simulink model "flexibleBeamILCBF"  (R2021a)
settings: Solver=ode23t  StartTime=0.0  StopTime=Tend  FixedStep=Ts  RelTol=1e-2
values from neighbouring files (symbols this model uses):
  G = G+2*(Cm(r)*Bm(r))/(s^2+2*zeta(r-1)*wn(r-1)*s+wn(r-1)^2)    [ModelFlexibleBeamFirstPrinciple.m]
  l = 500    [FRFSimscape.m]    (also in GPSnap.m; dataSetGPSnap_10092021.mat; dataSetGPSnap_10092021_2.mat)
  POI = 250    [FRFSimscape.m]
  Ts = 5e-4    (= 0.0005)    [FRFSimscape.m]    (also in GPSnap.m = 0.001; ILCBFSimscape.m = 0.001)
libraries: dspsrcs4 x2, simulink x1
settings Model: Creator=s152009  LastModifiedBy=s152009

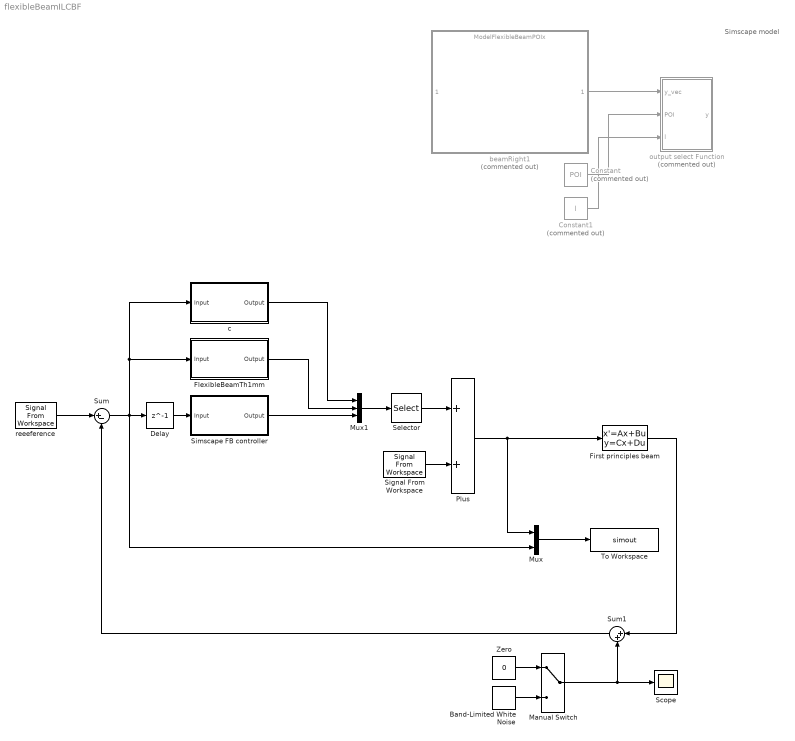
== system flexibleBeamILCBF ==
  note: Simscape model
  Band-Limited White Noise : simulink/Sources/Band-Limited White Noise  Cov=[1e-16]  Ts=Ts  seed=[23341]
  Constant : Constant  Commented=on  Value=POI
  Constant1 : Constant  Commented=on  Value=l
  Delay : Delay  DelayLength=1
  First principles beam : StateSpace  A=G.A  B=G.B  C=G.C  D=G.D  InitialCondition=0
  FlexibleBeamTh1mm : Subsystem
  Manual Switch : ManualSwitch
  Mux : Mux  Inputs=2
  Mux1 : Mux  Inputs=3
  Plus : Sum
  Scope : Scope
  Selector : Selector  InputPortWidth=3  IndexOptions=Index vector (dialog)  Indices=[1]  OutputSizes=1
  Signal From Workspace : dspsrcs4/Signal From Workspace  X=f_j  Ts=Ts  nsamps=1  OutputAfterFinalValue=Setting to zero  ignoreOrWarnInputAndFrameLengths=off  OutputFrames=off
  Simscape FB controller : Subsystem
  Sum : Sum  Inputs=|+-
  Sum1 : Sum  Inputs=|++
  To Workspace : ToWorkspace  VariableName=simout  SampleTime=Ts
  Zero : Constant  Value=0  OutDataTypeStr=Inherit: Inherit via back propagation
  beamRight1 : ModelReference  Commented=on  ModelNameDialog=ModelFlexibleBeamPOIx.slx  SimulationMode=Normal  ModelReferenceVersion=1.15
  c : Subsystem
  output select Function : MATLAB Function  Commented=on  TreatAsAtomicUnit=on
  reeeference : dspsrcs4/Signal From Workspace  X=r  Ts=Ts  nsamps=1  OutputAfterFinalValue=Holding final value  ignoreOrWarnInputAndFrameLengths=off  OutputFrames=off
  wires:
  reeeference/1 -> Sum/1
  Signal From Workspace/1 -> Plus/2
  Plus/1 -> First principles beam/1, Mux/1
  Sum/1 -> Mux/2, Delay/1, c/1(Input), FlexibleBeamTh1mm/1(Input)
  Mux/1 -> To Workspace/1
  Constant/1 -> output select Function/2(POI)
  Constant1/1 -> output select Function/3(l)
  Selector/1 -> Plus/1
  Simscape FB controller/1(Output) -> Mux1/3
  Delay/1 -> Simscape FB controller/1(Input)
  Mux1/1 -> Selector/1
  beamRight1/1 -> output select Function/1(y_vec)
  FlexibleBeamTh1mm/1(Output) -> Mux1/2
  First principles beam/1 -> Sum1/1
  Sum1/1 -> Sum/2
  Manual Switch/1 -> Scope/1, Sum1/2
  Zero/1 -> Manual Switch/1
  Band-Limited White Noise/1 -> Manual Switch/2
  c/1(Output) -> Mux1/1

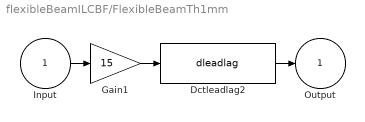
== system flexibleBeamILCBF/FlexibleBeamTh1mm ==
  Input : Inport
  Dctleadlag2 : S-Function  FunctionName=dleadlag  Parameters=f_num, f_den, 0.001  SFunctionDeploymentMode=off  EnableBusSupport=off  mask(dctools){f_num=0.5, f_den=5}
      mask prompts: f_num "Zero [Hz]"; f_den "Pole [Hz]"
      mask help: This block implements a discrete time leadlag filter.
      mask Display: disp('DCT leadlag')
  Gain1 : Gain  Gain=15
  Output : Outport
  wires:
  Input/1 -> Gain1/1
  Gain1/1 -> Dctleadlag2/1
  Dctleadlag2/1 -> Output/1

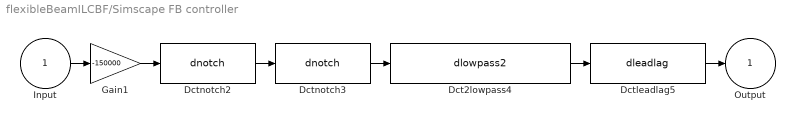
== system flexibleBeamILCBF/Simscape FB controller ==
  Input : Inport
  Dct2lowpass4 : S-Function  FunctionName=dlowpass2  Parameters=f_den, b_den, 0.001  SFunctionDeploymentMode=off  EnableBusSupport=off  mask(dctools){f_den=10, b_den=0.7}
      mask prompts: f_den "Pole [Hz]"; b_den "Damping pole [-]"
      mask help: This block implements a discrete time 2nd order lowpass filter.
      mask Display: disp('DCT 2nd order lowpass')
  Dctleadlag5 : S-Function  FunctionName=dleadlag  Parameters=f_num, f_den, 0.001  SFunctionDeploymentMode=off  EnableBusSupport=off  mask(dctools){f_num=45, f_den=405}
      mask prompts: f_num "Zero [Hz]"; f_den "Pole [Hz]"
      mask help: This block implements a discrete time leadlag filter.
      mask Display: disp('DCT leadlag')
  Dctnotch2 : S-Function  FunctionName=dnotch  Parameters=f_num, b_num, f_den, b_den, 0.001  SFunctionDeploymentMode=off  EnableBusSupport=off  mask(dctools){f_num=307, b_num=0.125, f_den=307, b_den=0.5}
      mask prompts: f_num "Zero [Hz]"; b_num "Damping zero [-]"; f_den "Pole [Hz]"; b_den "Damping pole [-]"
      mask help: This block implements a dicrete time 2nd order notch filter.
      mask Display: disp('DCT notch')
  Dctnotch3 : S-Function  FunctionName=dnotch  Parameters=f_num, b_num, f_den, b_den, 0.001  SFunctionDeploymentMode=off  EnableBusSupport=off  mask(dctools){f_num=61, b_num=0.15, f_den=61, b_den=0.5}
      mask prompts: f_num "Zero [Hz]"; b_num "Damping zero [-]"; f_den "Pole [Hz]"; b_den "Damping pole [-]"
      mask help: This block implements a dicrete time 2nd order notch filter.
      mask Display: disp('DCT notch')
  Gain1 : Gain  Gain=-150000
  Output : Outport
  wires:
  Input/1 -> Gain1/1
  Gain1/1 -> Dctnotch2/1
  Dctnotch2/1 -> Dctnotch3/1
  Dctnotch3/1 -> Dct2lowpass4/1
  Dct2lowpass4/1 -> Dctleadlag5/1
  Dctleadlag5/1 -> Output/1

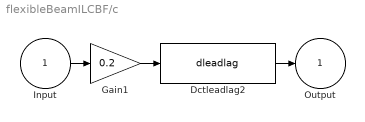
== system flexibleBeamILCBF/c ==
  Input : Inport
  Dctleadlag2 : S-Function  FunctionName=dleadlag  Parameters=f_num, f_den, 0.001  SFunctionDeploymentMode=off  EnableBusSupport=off  mask(dctools){f_num=0.5, f_den=5}
      mask prompts: f_num "Zero [Hz]"; f_den "Pole [Hz]"
      mask help: This block implements a discrete time leadlag filter.
      mask Display: disp('DCT leadlag')
  Gain1 : Gain  Gain=0.2
  Output : Outport
  wires:
  Dctleadlag2/1 -> Output/1
  Gain1/1 -> Dctleadlag2/1
  Input/1 -> Gain1/1

== matlab function flexibleBeamILCBF/output select Function ==
  data: y_vec input; y output; POI input; l input
function y = fcn(y_vec,POI,l)
if POI < l/2 && POI > 0 % left side poi
    y = y_vec(4);
elseif POI > l/2 && POI < l % right side poi
    y = y_vec(5);
elseif POI == l/2 % center poi
    y = y_vec(2);
elseif POI == 0 % left poi
    y = y_vec(1);
elseif POI == l % right poi
    y = y_vec(3);
else
    error('Not good POI measurement!')
end
end
